simulink model "HMI_C_S_28379D_FW"  (R2024b)
settings: Solver=ode4  StartTime=0.0  StopTime=Inf  FixedStep=Ts  RelTol=1e-3  EnableMultiTasking=on
InitFcn:
  | Ts=1e-4
model workspace (MAT data in the model file):
  encoderResolution = 2000
  hallOffset = '0.5'
  indexOffset = 850
  polePairs = '4'
libraries: simulink x4, c2837xDlib x2, c280xlib x2, c2802xlib x1
(part 2 of 2)

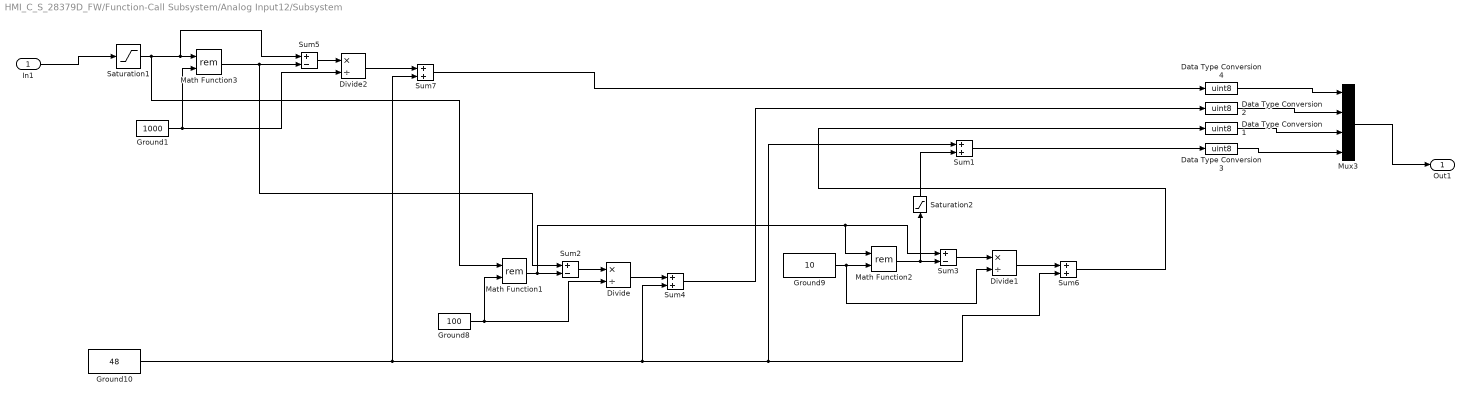
== system HMI_C_S_28379D_FW/Function-Call Subsystem/Analog Input12/Subsystem ==
  In1 : Inport
  Data Type Conversion{1..4} (4 alike) : DataTypeConversion  OutDataTypeStr=uint8  SaturateOnIntegerOverflow=off  RndMeth=Floor
  Divide : Product  Inputs=*/  OutDataTypeStr=int16
  Divide1 : Product  Inputs=*/  OutDataTypeStr=int16
  Divide2 : Product  Inputs=*/  OutDataTypeStr=int16
  Ground1 : Constant  Value=1000  OutDataTypeStr=int16
  Ground10 : Constant  Value=48  OutDataTypeStr=int16
  Ground8 : Constant  Value=100  OutDataTypeStr=int16
  Ground9 : Constant  Value=10  OutDataTypeStr=int16
  Math Function1 : Math  Operator=rem  SignedPower=on
  Math Function2 : Math  Operator=rem  SignedPower=on
  Math Function3 : Math  Operator=rem  SignedPower=on
  Mux3 : Mux
  Saturation1 : Saturate  UpperLimit=4095  LowerLimit=0  OutDataTypeStr=int16
  Saturation2 : Saturate  UpperLimit=9  LowerLimit=0
  Sum{1,4,6..7} (4 alike) : Sum  OutDataTypeStr=uint8
  Sum2 : Sum  Inputs=+-  OutDataTypeStr=double
  Sum3 : Sum  Inputs=+-
  Sum5 : Sum  Inputs=+-  OutDataTypeStr=double
  Out1 : Outport
  wires:
  Data Type Conversion2/1 -> Mux3/2
  Sum5/1 -> Divide2/1
  Ground10/1 -> Sum7/2, Sum4/2, Sum6/2, Sum1/1
  Math Function1/1 -> Sum2/2, Math Function2/1, Sum3/1
  Saturation1/1 -> Math Function1/1, Sum5/1, Math Function3/1
  Saturation2/1 -> Sum1/2
  In1/1 -> Saturation1/1
  Divide2/1 -> Sum7/1
  Data Type Conversion1/1 -> Mux3/3
  Sum4/1 -> Data Type Conversion2/1
  Math Function3/1 -> Sum2/1, Sum5/2
  Data Type Conversion4/1 -> Mux3/1
  Sum2/1 -> Divide/1
  Ground9/1 -> Divide1/2, Math Function2/2
  Sum6/1 -> Data Type Conversion1/1
  Ground8/1 -> Divide/2, Math Function1/2
  Ground1/1 -> Divide2/2, Math Function3/2
  Math Function2/1 -> Sum3/2, Saturation2/1
  Data Type Conversion3/1 -> Mux3/4
  Sum1/1 -> Data Type Conversion3/1
  Divide/1 -> Sum4/1
  Divide1/1 -> Sum6/1
  Sum7/1 -> Data Type Conversion4/1
  Sum3/1 -> Divide1/1
  Mux3/1 -> Out1/1
